simulink subsystem "aero_drag"  (R2025b)
settings: Solver=VariableStepAuto  StartTime=0.0  StopTime=10.0  RelTol=1e-3
libraries: nesl_utility x4, sm_lib x2, simlib_lib x1
settings Model: Creator=Dani  LastModifiedBy=Dani

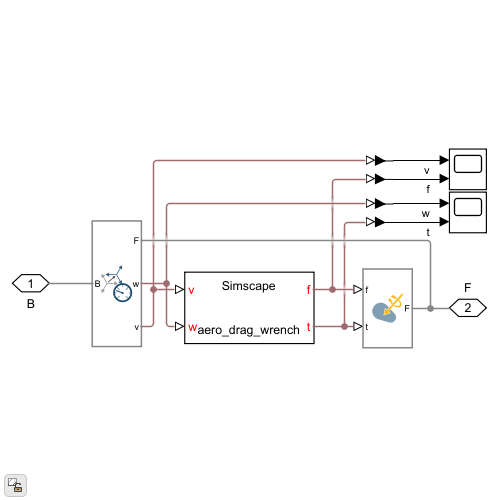
[thumbnail: Simulink's stored preview of the top-level diagram]
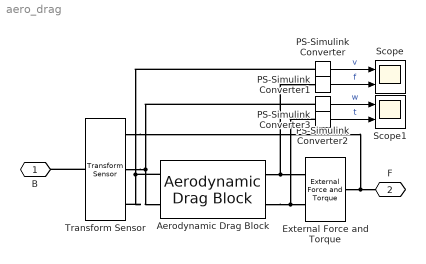
== system aero_drag ==
  Aerodynamic Drag Block : simlib_lib/aero/Aerodynamic Drag Block  D=[.5, 0, 0; 0, .8, 0; 0, 0, 1.2] N*s^2/m^2
      settings: InternalSimscapePortConfiguration="{\"Bottom\":[],\"Left\":[{\"id\":\"v\",\"label\":\"v\",\"type\":\"input\"},{\"id\":\"w\",\"label\":\"w\",\"type\":\"input\"}],\"Right\":[{\"id\":\"f\",\"label\":\"f\",\"type\":\"output\"},{\"id\":\"t\",\"label\":\"t\",\"type\":\"output\"}],\"Top\":[]}"
  External Force and Torque : sm_lib/Forces and Torques/External Force and Torque  EnableForceX=off  EnableForceY=off  EnableForceZ=off  EnableForce=on  ForceResolutionFrame=AttachedFrame  EnableTorqueX=off  EnableTorqueY=off  EnableTorqueZ=off  EnableTorque=on  TorqueResolutionFrame=AttachedFrame
  PS-Simulink Converter{,1..3} (4 alike) : nesl_utility/PS-Simulink Converter  PhysicalDomain=network_engine_domain  SubClassName=ps_output  LeftPortType=input  RightPortType=output  PseudoPeriodic=off  Frequencies=[]  VectorFormat=inherit  Unit=inherit  AffineConversion=off
  Scope : Scope  NumInputPorts=2
      settings: ActiveDisplayYMinimum=-2.5217605006062391  ActiveDisplayYMaximum=1.4068168123378904
  Scope1 : Scope  NumInputPorts=2
      settings: ActiveDisplayYMinimum=-2.5217605006062391  ActiveDisplayYMaximum=1.4068168123378904
  Transform Sensor : sm_lib/Frames and Transforms/Transform Sensor  MeasurementFrame=Follower  RotationSequence=XYX  SenseAngle=off  SenseAxis=off  SenseQ=off  SenseR=off  SenseRotationSequence=off  SenseOmegaX=off  SenseOmegaY=off  SenseOmegaZ=off  SenseOmega=on  SenseQDot=off  SenseRDot=off  SenseRotationSequenceDot=off  SenseAlphaX=off  SenseAlphaY=off  SenseAlphaZ=off  SenseAlpha=off  SenseQDDot=off  SenseRDDot=off  SenseX=off  SenseY=off  SenseZ=off  SenseXYZ=off  SenseRad=off  SenseAzim=off  SenseDist=off  SenseInc=off  SenseXDot=off  SenseYDot=off  SenseZDot=off  SenseXYZDot=on  SenseRadDot=off  SenseAzimDot=off  SenseDistDot=off  SenseIncDot=off  SenseXDDot=off  SenseYDDot=off  SenseZDDot=off  SenseXYZDDot=off  SenseRadDDot=off  SenseAzimDDot=off  SenseDistDDot=off  SenseIncDDot=off
  B : PMIOPort  Side=Left
  F : PMIOPort  Port=2  Side=Right
  wires:
  PS-Simulink Converter/1 -> Scope/1  "v"
  PS-Simulink Converter1/1 -> Scope/2  "f"
  PS-Simulink Converter2/1 -> Scope1/1  "w"
  PS-Simulink Converter3/1 -> Scope1/2  "t"
  connections:
  Transform Sensor/RConn3 -- Aerodynamic Drag Block/LConn1 -- PS-Simulink Converter/LConn1
  PS-Simulink Converter1/LConn1 -- External Force and Torque/LConn1 -- Aerodynamic Drag Block/RConn1
  Transform Sensor/RConn1 -- F/RConn1 -- External Force and Torque/RConn1
  Aerodynamic Drag Block/RConn2 -- External Force and Torque/LConn2 -- PS-Simulink Converter3/LConn1
  Transform Sensor/RConn2 -- Aerodynamic Drag Block/LConn2 -- PS-Simulink Converter2/LConn1
  Transform Sensor/LConn1 -- B/RConn1
